simulink subsystem "sun_sensor_model"  (R2024a)
settings: Solver=VariableStepAuto  StartTime=0.0  StopTime=10.0  RelTol=1e-3
settings Model: Creator=joshu  LastModifiedBy=joshu

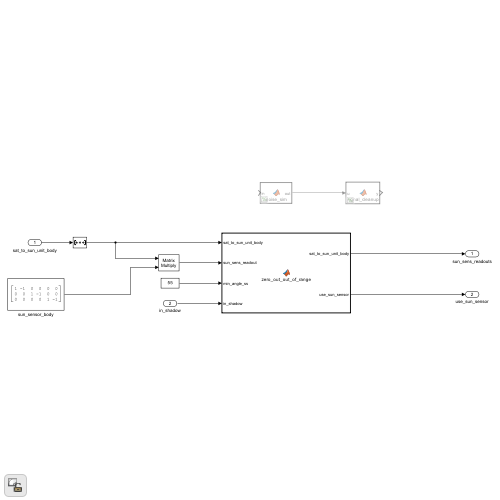
[thumbnail: Simulink's stored preview of the top-level diagram]
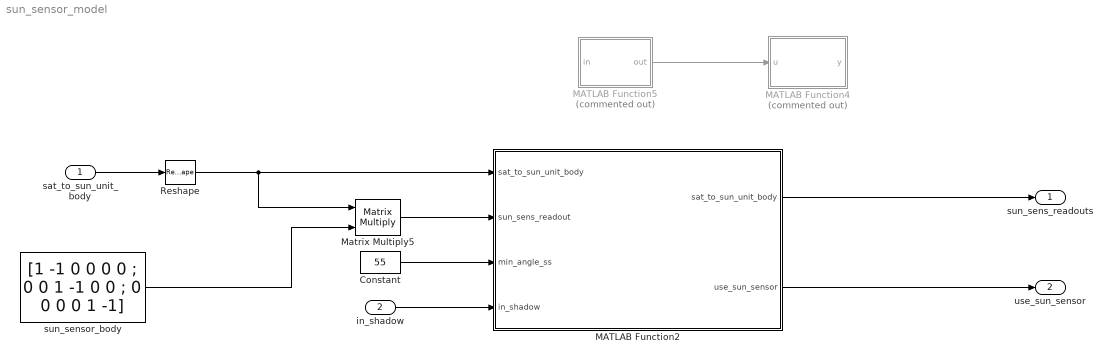
== system sun_sensor_model ==
  sat_to_sun_unit_body : Inport
  in_shadow : Inport  Port=2
  Constant : Constant  Value=55
  MATLAB Function2 : MATLAB Function  TreatAsAtomicUnit=on
  MATLAB Function4 : MATLAB Function  Commented=on  TreatAsAtomicUnit=on
  MATLAB Function5 : MATLAB Function  Commented=on  TreatAsAtomicUnit=on
  Matrix Multiply5 : Product  Multiplication=Matrix(*)
  Reshape : Reshape  OutputDimensionality=Row vector (2-D)
  sun_sensor_body : Constant  Value=[1 -1 0 0 0 0 ; 0 0 1 -1 0 0 ; 0 0 0 0 1 -1]
  sun_sens_readouts : Outport
  use_sun_sensor : Outport  Port=2
  wires:
  Constant/1 -> MATLAB Function2/3(min_angle_ss)
  MATLAB Function2/1(sat_to_sun_unit_body) -> sun_sens_readouts/1
  sun_sensor_body/1 -> Matrix Multiply5/2
  Matrix Multiply5/1 -> MATLAB Function2/2(sun_sens_readout)
  sat_to_sun_unit_body/1 -> Reshape/1
  Reshape/1 -> MATLAB Function2/1("sat_to_sun_unit_body "), Matrix Multiply5/1
  in_shadow/1 -> MATLAB Function2/4(in_shadow)
  MATLAB Function5/1(out) -> MATLAB Function4/1(u)
  MATLAB Function2/2(use_sun_sensor) -> use_sun_sensor/1

== matlab function sun_sensor_model/MATLAB Function2 ==
  data: sat_to_sun_unit_body output; sat_to_sun_unit_body input; sun_sens_readout input; use_sun_sensor output; min_angle_ss input; in_shadow input
function [sat_to_sun_unit_body,use_sun_sensor] = zero_out_out_of_range(sat_to_sun_unit_body, sun_sens_readout, min_angle_ss, in_shadow)
    
    min_value = cosd(min_angle_ss);
    out = sun_sens_readout;
    for i = 1:length(out)
        if out(i) < min_value
            out(i) = 0;
        end
    end
    
    use_sun_sensor = ((sum(out) ~= 0) & ~in_shadow);

    if use_sun_sensor
        %sat_to_sun_unit_body = sat_to_sun_unit_body;
    else
        sat_to_sun_unit_body = zeros(1,3);
    end

== matlab function sun_sensor_model/MATLAB Function4 ==
  data: u input; y output
function y = signal_cleanup(u)
y = [0,0,0];

if u(1) == 0
    y(1) = -u(2);
else
    y(1) = u(1);
end

if u(3) == 0
    y(2) = -u(4);
else
    y(2) = u(3);
end

if u(5) == 0
    y(3) = -u(6);
else
    y(3) = u(5);
end


end

== matlab function sun_sensor_model/MATLAB Function5 ==
  settings: updateMethod=DISCRETE
  data: in input; out output
function out = noise_sim(in)

    out = in;

    for i = 1:length(out)
        sgn = sign(out(i));
        ang = acosd(abs(out(i)));
        if ang <= 45
            %out(i) = cosd(ang + (rand()*0.6-0.3))*sgn;
        elseif ang <= 60
            %out(i) = cosd(ang + (rand()*1.2-0.6))*sgn;
        end
    end
